simulink model "GRIPPER_TEST"  (R2015b)
settings: Solver=VariableStepAuto  StartTime=0.0  StopTime=inf  RelTol=1e-3
undefined symbols (not defined in the file): Position, Position_SL_Info
libraries: robotlib x3
settings Model: Creator=daniele  LastModifiedBy=daniele

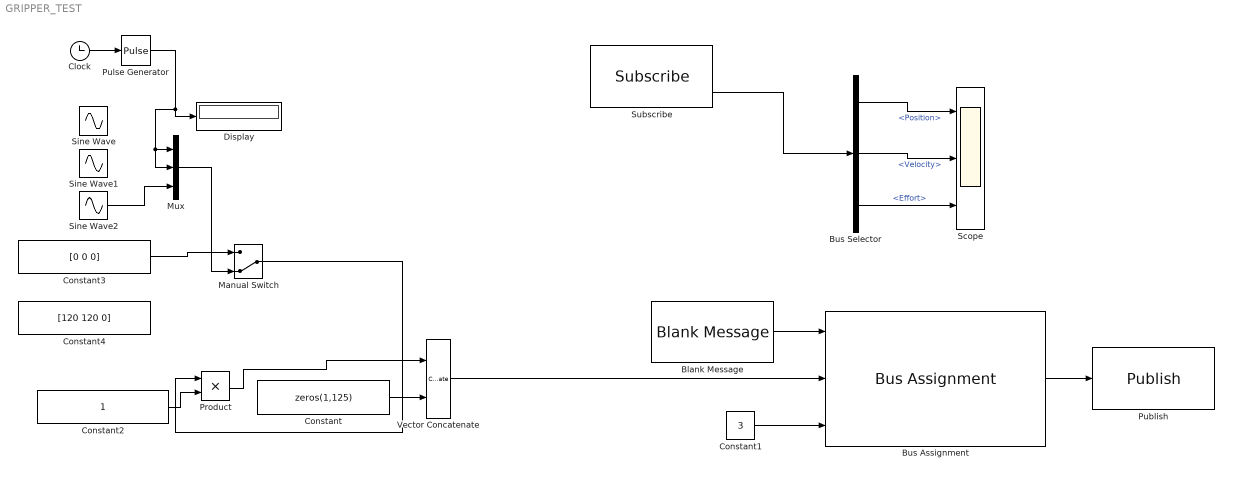
== system GRIPPER_TEST ==
  Blank Message : robotlib/Blank Message  SourceLibraryInfo=This block requires Robotics System Toolbox  messageType=sensor_msgs/JointState  SampleTime=inf
  Bus Assignment : BusAssignment  AssignedSignals=Position,Position_SL_Info.CurrentLength
  Bus Selector : BusSelector  OutputSignals=Position,Velocity,Effort
  Clock : Clock
  Constant : Constant  Value=zeros(1,125)
  Constant1 : Constant  Value=3  OutDataTypeStr=uint32
  Constant2 : Constant
  Constant3 : Constant  Value=[0 0 0]
  Constant4 : Constant  Value=[120 120 0]
  Display : Display
  Manual Switch : ManualSwitch  CurrentSetting=0
  Mux : Mux  Inputs=3
  Product : Product
  Publish : robotlib/Publish  SourceLibraryInfo=This block requires Robotics System Toolbox  topicSource=Select from ROS network  topic=/trifinger2/joint_command  messageType=sensor_msgs/JointState  messageQueueLength=1
  Pulse Generator : DiscretePulseGenerator  PulseType=Time based  TimeSource=Use external signal  Amplitude=90  Period=500  PulseWidth=50
  Scope : Scope  NumInputPorts=3
  Sine Wave : Sin  Amplitude=45  Bias=45  Frequency=0.01  SampleTime=0
  Sine Wave1 : Sin  Amplitude=45  Bias=45  Frequency=0.01  SampleTime=0
  Sine Wave2 : Sin  Amplitude=0  SampleTime=0
  Subscribe : robotlib/Subscribe  SourceLibraryInfo=This block requires Robotics System Toolbox  topicSource=Select from ROS network  topic=/trifinger2/joint_state  messageType=sensor_msgs/JointState  sampleTime=-1  messageQueueLength=1
  Vector Concatenate : Concatenate
  wires:
  Bus Assignment/1 -> Publish/1
  Constant1/1 -> Bus Assignment/3
  Vector Concatenate/1 -> Bus Assignment/2
  Blank Message/1 -> Bus Assignment/1
  Constant/1 -> Vector Concatenate/2
  Constant2/1 -> Product/2
  Product/1 -> Vector Concatenate/1
  Constant3/1 -> Manual Switch/1
  Manual Switch/1 -> Product/1
  Sine Wave2/1 -> Mux/3
  Clock/1 -> Pulse Generator/1
  Pulse Generator/1 -> Mux/1, Mux/2, Display/1
  Mux/1 -> Manual Switch/2
  Subscribe/2 -> Bus Selector/1
  Bus Selector/2 -> Scope/2  "<Velocity>"
  Bus Selector/1 -> Scope/1  "<Position>"
  Bus Selector/3 -> Scope/3  "<Effort>"
